simulink model "Tp1"  (R2019a)
settings: Solver=VariableStepAuto  StartTime=0.0  StopTime=5  MaxStep=0.01  RelTol=1e-3
settings Model: Creator=valen  LastModifiedBy=User
settings DataIOCC: ReturnWorkspaceOutputs=off
settings DebuggingCC: PregeneratedLibrarySubsystemCodeDiagnostic=none  ArithmeticOperatorsInVariantConditions=warning
settings SFSimCC: SimUseLocalCustomCode=off
settings RTWCC: RTWUseLocalCustomCode=off

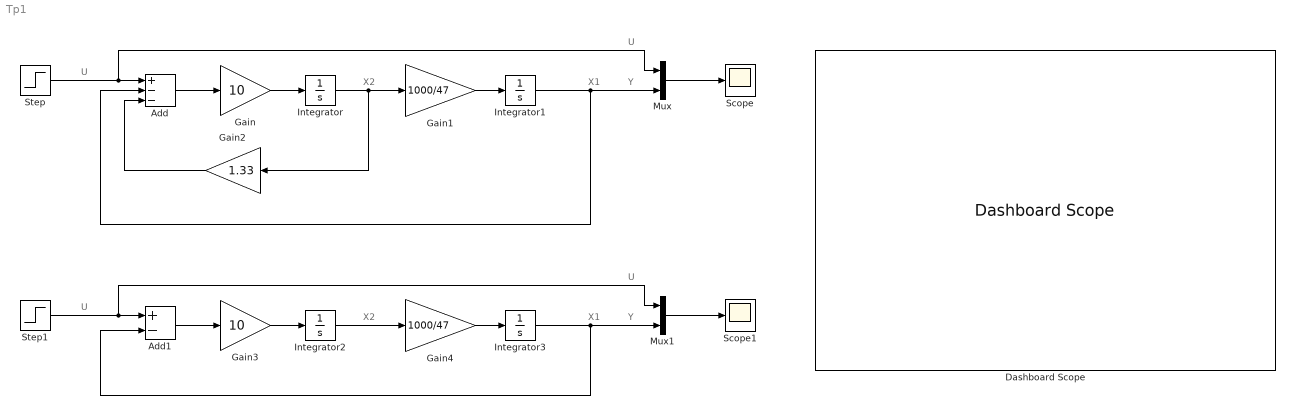
== system Tp1 ==
  note: X2
  note: U
  note: U
  note: X2
  note: X1
  note: X1
  note: Y
  note: Y
  note: U
  note: U
  Add : Sum  Inputs=+--
  Add1 : Sum  Inputs=+-
  Dashboard Scope : DashboardScope
  Gain : Gain  Gain=10
  Gain1 : Gain  Gain=1000/47
  Gain2 : Gain  Gain=1.33
  Gain3 : Gain  Gain=10
  Gain4 : Gain  Gain=1000/47
  Integrator{,1..3} (4 alike) : Integrator
  Mux : Mux  Inputs=2
  Mux1 : Mux  Inputs=2
  Scope : Scope
  Scope1 : Scope
  Step : Step  SampleTime=0
  Step1 : Step  SampleTime=0
  wires:
  Gain/1 -> Integrator/1
  Step/1 -> Mux/1, Add/1
  Add/1 -> Gain/1
  Gain1/1 -> Integrator1/1
  Integrator1/1 -> Add/2, Mux/2
  Integrator/1 -> Gain1/1, Gain2/1
  Mux/1 -> Scope/1
  Gain2/1 -> Add/3
  Gain3/1 -> Integrator2/1
  Step1/1 -> Mux1/1, Add1/1
  Gain4/1 -> Integrator3/1
  Integrator3/1 -> Add1/2, Mux1/2
  Integrator2/1 -> Gain4/1
  Add1/1 -> Gain3/1
  Mux1/1 -> Scope1/1
